simulink model "ATSS_Plausability"  (R2024b)
settings: Solver=VariableStepAuto  StartTime=0.0  StopTime=11  RelTol=1e-3
libraries: simulink x1
settings Model: Creator=Michele  LastModifiedBy=feder
settings ConfigComp: CovMetricSettings=dcmwe

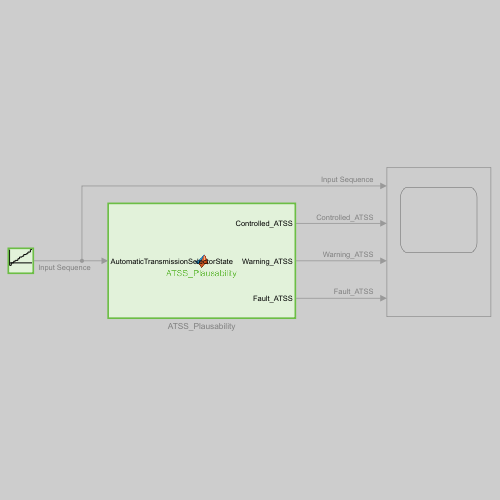
[thumbnail: Simulink's stored preview of the top-level diagram]
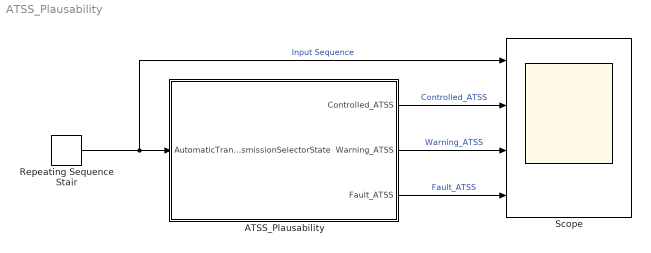
== system ATSS_Plausability ==
  ATSS_Plausability : MATLAB Function  TreatAsAtomicUnit=on
  Repeating Sequence Stair : simulink/Sources/Repeating Sequence Stair  OutValues=[-1 0 0.5 1 1.5 2 2.5 3 3.5 4 5].'  tsamp=1  OutMin=[]  OutMax=[]  OutDataTypeStr=single  OutputDataTypeScalingMode=single  OutDataType=Enum: TransmissionState  ConRadixGroup=Best Precision: Vector-wise  OutScaling=[]
  Scope : Scope  NumInputPorts=4
  wires:
  ATSS_Plausability/1(Controlled_ATSS) -> Scope/2  "Controlled_ATSS"
  ATSS_Plausability/3(Fault_ATSS) -> Scope/4  "Fault_ATSS"
  ATSS_Plausability/2(Warning_ATSS) -> Scope/3  "Warning_ATSS"
  Repeating Sequence Stair/1 -> Scope/1, ATSS_Plausability/1(AutomaticTransmissionSelectorState)  "Input Sequence"

== matlab function ATSS_Plausability/ATSS_Plausability ==
  data: AutomaticTransmissionSelectorState input; Controlled_ATSS output Enum: TransmissionState; Warning_ATSS output Enum: WarningType; Fault_ATSS output
function [Controlled_ATSS,Warning_ATSS,Fault_ATSS] = ATSS_Plausability(AutomaticTransmissionSelectorState)

Controlled_ATSS = TransmissionState(2);
Warning_ATSS = WarningType(0);
Fault_ATSS = boolean(0);

ValidModes = [0 1 2 3 4];

if any(AutomaticTransmissionSelectorState == ValidModes)

    Controlled_ATSS = TransmissionState(AutomaticTransmissionSelectorState);
    
else

    Warning_ATSS = WarningType(2);
    Fault_ATSS = boolean(1);

end
